simulink model "UAV_UGV_Coop"  (R2026a)
settings: Solver=ode4  StopTime=650  FixedStep=1e-3  MaxStep=0.001  MinStep=1e-6
PreLoadFcn:
  | % Caricamento automatico di tutte le variabili salvate
  | 
  | load('MappaEdifici.mat');
  | load('WaypointData.mat');
  | load('MappaGroundTruth.mat');
  | load('MappaScoperta_Altis.mat');
  | load('Percoso_UGV.mat');
  | load('UAV_x_d.mat');
  | load('UAV_x_r.mat');
  | load('UAV_y_d.mat');
  | load('UAV_y_r.mat');
  | load('UAV_z_d.mat');
  | load('UAV_z_r.mat');
  | load('UAV_phi_d.mat');
  | load('UAV_phi_r.mat');
  | load('UAV_theta_d.mat');
  | load('UAV_theta_r.mat');
  | load('UGV_x_d.mat');
  | load('UGV_x_r.mat');
  | load('UGV_y_d.mat');
  | load('UGV_y_r.mat');
  | load('UGV_psi.mat');
  | load('UGV_theta.mat');
  | load('A_fov.mat');
  | load('tout.mat');
model workspace: external: MAT-File MappaGroundTruth.mat (data not in the file)
undefined symbols (not defined in the file): MAPPA_EDIFICI, MAPPA_GROUND_TRUTH
settings Model: Creator=adriano  LastModifiedBy=Salvatore

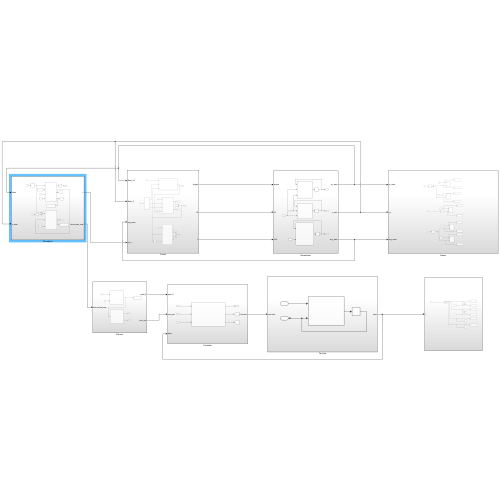
[thumbnail: Simulink's stored preview of the top-level diagram]
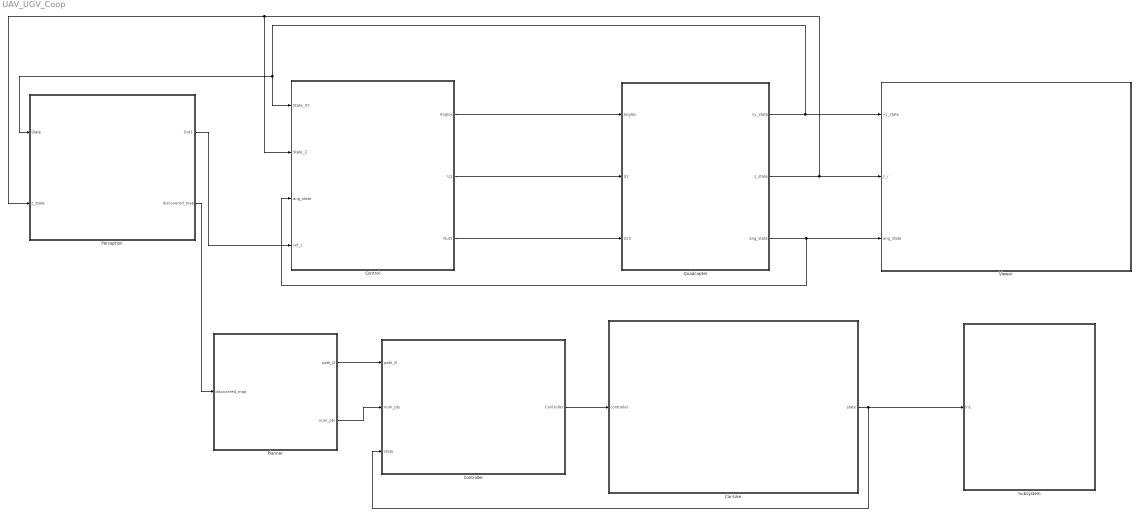
== system UAV_UGV_Coop ==
  Car-Like : Subsystem
  Control : Subsystem
  Controller : Subsystem
  Perception : Subsystem
  Planner : Subsystem
  Quadcopter : Subsystem
  Subsystem : Subsystem
  Viewer : Subsystem
  wires:
  Quadcopter/2(z_state) -> Control/2(State_Z), Perception/2(z_state), Viewer/2(z_r)
  Perception/1(Out1) -> Control/4(ref_z)
  Quadcopter/1(xy_state) -> Control/1(State_XY), Perception/1(State), Viewer/1(xy_state)
  Control/2(U1) -> Quadcopter/2(U1)
  Quadcopter/3(ang_state) -> Viewer/3(ang_state), Control/3(ang_state)
  Control/1(Angles) -> Quadcopter/1(angles)
  Control/3(Out1) -> Quadcopter/3(U23)
  Perception/2(discovered_map) -> Planner/1(discovered_map)
  Planner/1(path_D) -> Controller/1(path_D)
  Planner/2(num_pts) -> Controller/2(num_pts)
  Controller/1(Controller) -> Car-Like/1(controller)
  Car-Like/1(state) -> Controller/3(state), Subsystem/1(In1)

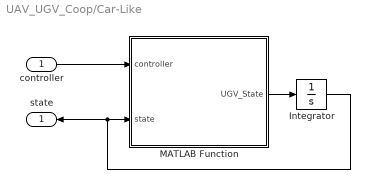
== system UAV_UGV_Coop/Car-Like ==
  controller : Inport
  Integrator : Integrator  InitialCondition=[17.0; 155.0; 0.0; 0.0]
  MATLAB Function : MATLAB Function  TreatAsAtomicUnit=on
  state : Outport
  wires:
  MATLAB Function/1(UGV_State) -> Integrator/1
  Integrator/1 -> MATLAB Function/2(state), state/1
  controller/1 -> MATLAB Function/1(controller)

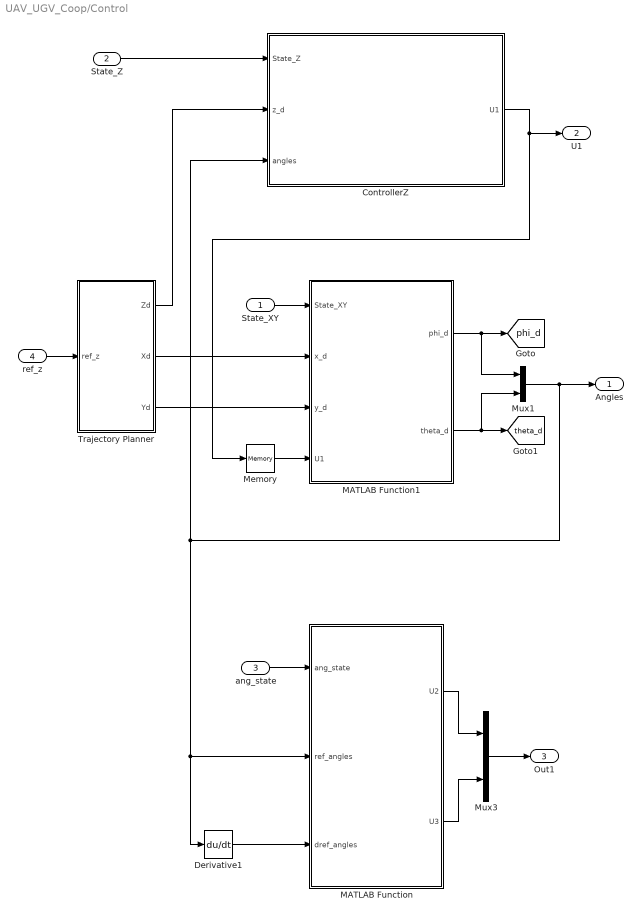
== system UAV_UGV_Coop/Control ==
  State_XY : Inport
  State_Z : Inport  Port=2
  ang_state : Inport  Port=3
  ref_z : Inport  Port=4
  ControllerZ : Subsystem
  Derivative1 : Derivative
  MATLAB Function : MATLAB Function  TreatAsAtomicUnit=on
  MATLAB Function1 : MATLAB Function  TreatAsAtomicUnit=on
  Memory : Memory
  Mux1 : Mux  Inputs=2
  Mux3 : Mux  Inputs=2
  Trajectory Planner : Subsystem
  Angles : Outport
  U1 : Outport  Port=2
  Out1 : Outport  Port=3
  tag scope: phi_d=global, theta_d=global
  wires:
  ref_z/1 -> Trajectory Planner/1(ref_z)
  State_Z/1 -> ControllerZ/1(State_Z)
  Trajectory Planner/1(Zd) -> ControllerZ/2(z_d)
  ControllerZ/1(U1) -> U1/1, Memory/1
  State_XY/1 -> MATLAB Function1/1(State_XY)
  ang_state/1 -> MATLAB Function/1(ang_state)
  Mux1/1 -> ControllerZ/3(angles), MATLAB Function/2(ref_angles), Derivative1/1, Angles/1
  MATLAB Function/1(U2) -> Mux3/1
  MATLAB Function/2(U3) -> Mux3/2
  Mux3/1 -> Out1/1
  Memory/1 -> MATLAB Function1/4(U1)
  MATLAB Function1/2(theta_d) -> [theta_d], Mux1/2
  MATLAB Function1/1(phi_d) -> [phi_d], Mux1/1
  Derivative1/1 -> MATLAB Function/3(dref_angles)
  Trajectory Planner/2(Xd) -> MATLAB Function1/2(x_d)
  Trajectory Planner/3(Yd) -> MATLAB Function1/3(y_d)

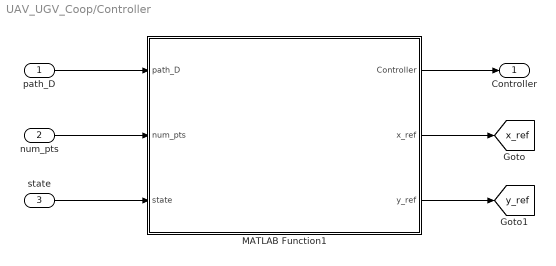
== system UAV_UGV_Coop/Controller ==
  path_D : Inport
  num_pts : Inport  Port=2
  state : Inport  Port=3
  MATLAB Function1 : MATLAB Function  TreatAsAtomicUnit=on
  Controller : Outport
  tag scope: x_ref=global, y_ref=global
  wires:
  state/1 -> MATLAB Function1/3(state)
  path_D/1 -> MATLAB Function1/1(path_D)
  MATLAB Function1/1(Controller) -> Controller/1
  num_pts/1 -> MATLAB Function1/2(num_pts)
  MATLAB Function1/2(x_ref) -> [x_ref]
  MATLAB Function1/3(y_ref) -> [y_ref]

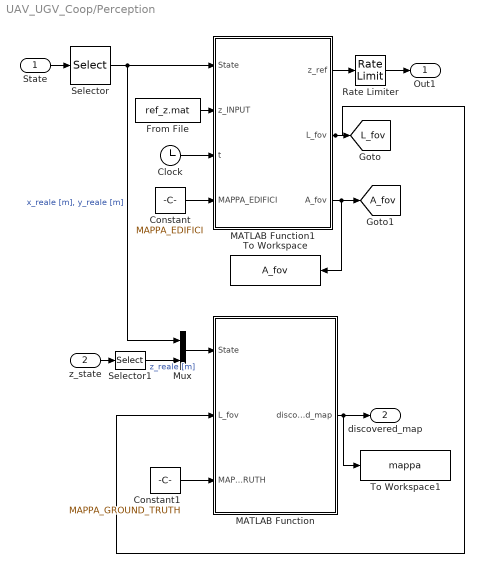
== system UAV_UGV_Coop/Perception ==
  State : Inport
  z_state : Inport  Port=2
  Clock : Clock
  Constant : Constant  Value=MAPPA_EDIFICI
  Constant1 : Constant  Value=MAPPA_GROUND_TRUTH
  From File : FromFile  FileName=ref_z.mat  SampleTime=0
  MATLAB Function : MATLAB Function  TreatAsAtomicUnit=on
  MATLAB Function1 : MATLAB Function  TreatAsAtomicUnit=on
  Mux : Mux  Inputs=2
  Rate Limiter : RateLimiter  SampleTimeMode=inherited
  Selector : Selector  InputPortWidth=4  IndexOptions=Index vector (dialog)  Indices=[1 3]  OutputSizes=1
  Selector1 : Selector  InputPortWidth=2  IndexOptions=Index vector (dialog)  Indices=[1]  OutputSizes=1
  To Workspace : ToWorkspace  VariableName=A_fov  SaveFormat=Timeseries  SampleTime=-1
  To Workspace1 : ToWorkspace  VariableName=mappa  SaveFormat=Timeseries  SampleTime=-1
      settings: MaxDataPoints=1
  Out1 : Outport
  discovered_map : Outport  Port=2
  tag scope: A_fov=global, L_fov=global
  wires:
  MATLAB Function1/2(L_fov) -> MATLAB Function/2(L_fov), [L_fov]
  From File/1 -> MATLAB Function1/2(z_INPUT)
  Rate Limiter/1 -> Out1/1
  MATLAB Function1/3(A_fov) -> [A_fov], To Workspace/1
  MATLAB Function1/1(z_ref) -> Rate Limiter/1
  State/1 -> Selector/1
  Selector/1 -> MATLAB Function1/1(State), Mux/1  "x_reale [m], y_reale [m]"
  Clock/1 -> MATLAB Function1/3(t)
  Constant/1 -> MATLAB Function1/4(MAPPA_EDIFICI)
  z_state/1 -> Selector1/1
  Selector1/1 -> Mux/2  "z_reale [m]"
  Mux/1 -> MATLAB Function/1(State)
  Constant1/1 -> MATLAB Function/3(MAPPA_GROUND_TRUTH)
  MATLAB Function/1(discovered_map) -> To Workspace1/1, discovered_map/1

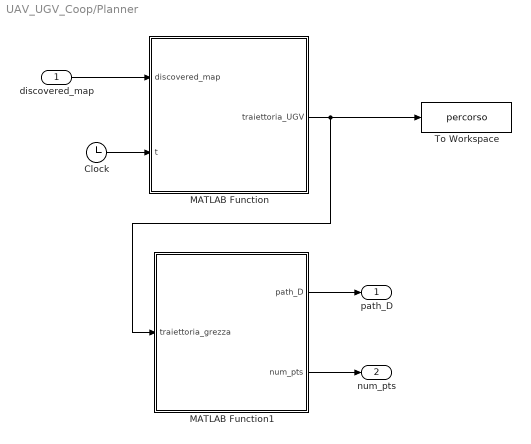
== system UAV_UGV_Coop/Planner ==
  discovered_map : Inport
  Clock : Clock
  MATLAB Function : MATLAB Function  TreatAsAtomicUnit=on
  MATLAB Function1 : MATLAB Function  TreatAsAtomicUnit=on
  To Workspace : ToWorkspace  VariableName=percorso  SaveFormat=Timeseries  SampleTime=-1
      settings: MaxDataPoints=1
  path_D : Outport
  num_pts : Outport  Port=2
  wires:
  Clock/1 -> MATLAB Function/2(t)
  MATLAB Function/1(traiettoria_UGV) -> To Workspace/1, MATLAB Function1/1(traiettoria_grezza)
  discovered_map/1 -> MATLAB Function/1(discovered_map)
  MATLAB Function1/1(path_D) -> path_D/1
  MATLAB Function1/2(num_pts) -> num_pts/1

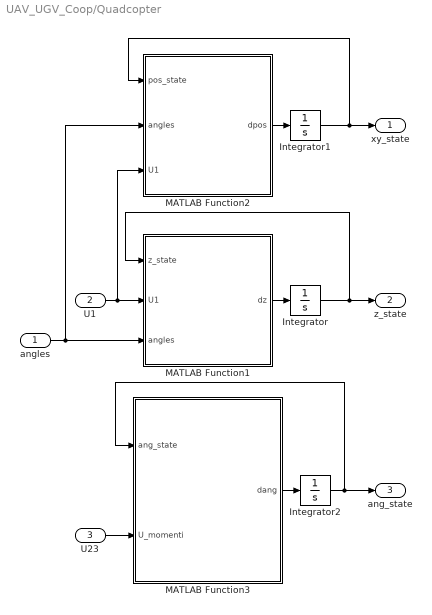
== system UAV_UGV_Coop/Quadcopter ==
  angles : Inport
  U1 : Inport  Port=2
  U23 : Inport  Port=3
  Integrator : Integrator
  Integrator1 : Integrator
  Integrator2 : Integrator
  MATLAB Function1 : MATLAB Function  TreatAsAtomicUnit=on
  MATLAB Function2 : MATLAB Function  TreatAsAtomicUnit=on
  MATLAB Function3 : MATLAB Function  TreatAsAtomicUnit=on
  xy_state : Outport
  z_state : Outport  Port=2
  ang_state : Outport  Port=3
  wires:
  MATLAB Function1/1(dz) -> Integrator/1
  Integrator/1 -> z_state/1, MATLAB Function1/1(z_state)
  angles/1 -> MATLAB Function2/2(angles), MATLAB Function1/3(angles)
  MATLAB Function2/1(dpos) -> Integrator1/1
  Integrator1/1 -> MATLAB Function2/1(pos_state), xy_state/1
  U1/1 -> MATLAB Function1/2(U1), MATLAB Function2/3(U1)
  MATLAB Function3/1(dang) -> Integrator2/1
  Integrator2/1 -> ang_state/1, MATLAB Function3/1(ang_state)
  U23/1 -> MATLAB Function3/2(U_momenti)

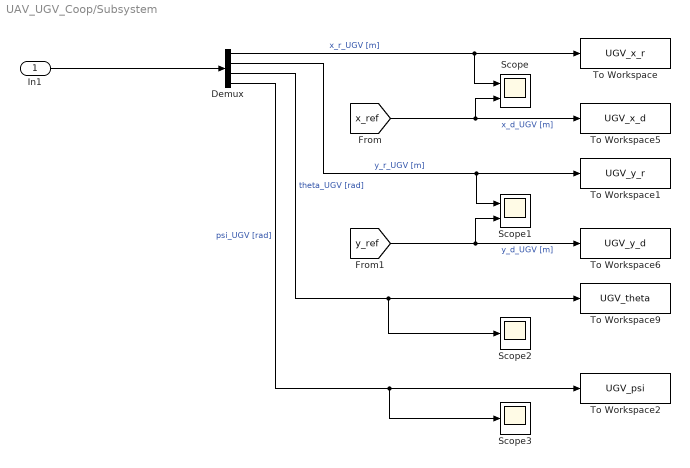
== system UAV_UGV_Coop/Subsystem ==
  In1 : Inport
  Demux : Demux
  Scope : Scope  NumInputPorts=2
      settings: ActiveDisplayYMinimum=-148.99376559580284  ActiveDisplayYMaximum=93.973074247656058  DataLoggingVariableName=ScopeData3
  Scope1 : Scope  NumInputPorts=2
      settings: ActiveDisplayYMinimum=31.631627910476041  ActiveDisplayYMaximum=174.01442830668728  DataLoggingVariableName=ScopeData4
  Scope2 : Scope
      settings: ActiveDisplayYMinimum=-4.4152539279638745  ActiveDisplayYMaximum=4.7250316272107744  DataLoggingVariableName=ScopeData5
  Scope3 : Scope
      settings: ActiveDisplayYMinimum=-0.76358154774750753  ActiveDisplayYMaximum=0.76358154774750753  DataLoggingVariableName=ScopeData6
  To Workspace : ToWorkspace  VariableName=UGV_x_r  SaveFormat=Timeseries  SampleTime=-1
  To Workspace1 : ToWorkspace  VariableName=UGV_y_r  SaveFormat=Timeseries  SampleTime=-1
  To Workspace2 : ToWorkspace  VariableName=UGV_psi  SaveFormat=Timeseries  SampleTime=-1
  To Workspace5 : ToWorkspace  VariableName=UGV_x_d  SaveFormat=Timeseries  SampleTime=-1
  To Workspace6 : ToWorkspace  VariableName=UGV_y_d  SaveFormat=Timeseries  SampleTime=-1
  To Workspace9 : ToWorkspace  VariableName=UGV_theta  SaveFormat=Timeseries  SampleTime=-1
  wires:
  Demux/2 -> Scope1/1, To Workspace1/1  "y_r_UGV [m]"
  Demux/1 -> Scope/1, To Workspace/1  "x_r_UGV [m]"
  [x_ref] -> Scope/2, To Workspace5/1  "x_d_UGV [m]"
  In1/1 -> Demux/1
  [y_ref] -> To Workspace6/1, Scope1/2  "y_d_UGV [m]"
  Demux/3 -> To Workspace9/1, Scope2/1  "theta_UGV [rad]"
  Demux/4 -> To Workspace2/1, Scope3/1  "psi_UGV [rad]"

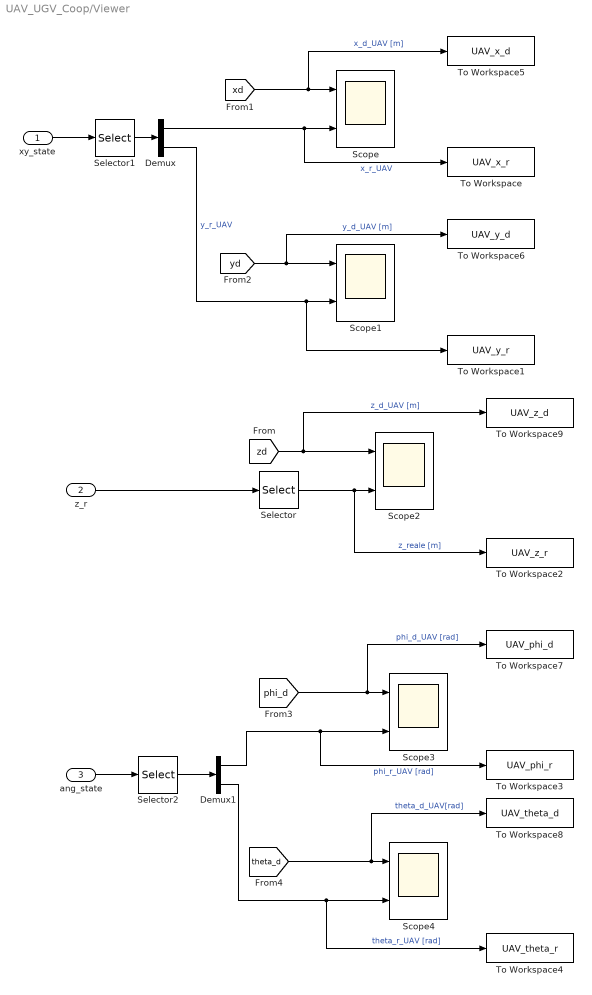
== system UAV_UGV_Coop/Viewer ==
  xy_state : Inport
  z_r : Inport  Port=2
  ang_state : Inport  Port=3
  Demux : Demux  Outputs=2
  Demux1 : Demux  Outputs=2
  Scope{,1..4} (5 alike) : Scope  NumInputPorts=2
      Scope settings: ActiveDisplayYMinimum=-242.12221615870175  ActiveDisplayYMaximum=120.41682539227989
      Scope1 settings: ActiveDisplayYMinimum=-23.676037505376105  ActiveDisplayYMaximum=207.37773635103918
      Scope2 settings: ActiveDisplayYMinimum=-7.8867312001852117  ActiveDisplayYMaximum=70.963722945541591  DataLoggingVariableName=ScopeData2
      Scope3 settings: ActiveDisplayYMinimum=-0.83331111959754556  ActiveDisplayYMaximum=0.72502273318878152  DataLoggingVariableName=ScopeData7
      Scope4 settings: ActiveDisplayYMinimum=-1  ActiveDisplayYMaximum=1  DataLoggingVariableName=ScopeData8
  Selector : Selector  InputPortWidth=2  IndexOptions=Index vector (dialog)  Indices=[1]  OutputSizes=1
  Selector1 : Selector  InputPortWidth=4  IndexOptions=Index vector (dialog)  Indices=[1 3]  OutputSizes=1
  Selector2 : Selector  InputPortWidth=4  IndexOptions=Index vector (dialog)  Indices=[1 3]  OutputSizes=1
  To Workspace : ToWorkspace  VariableName=UAV_x_r  SaveFormat=Timeseries  SampleTime=-1
  To Workspace1 : ToWorkspace  VariableName=UAV_y_r  SaveFormat=Timeseries  SampleTime=-1
  To Workspace2 : ToWorkspace  VariableName=UAV_z_r  SaveFormat=Timeseries  SampleTime=-1
  To Workspace3 : ToWorkspace  VariableName=UAV_phi_r  SaveFormat=Timeseries  SampleTime=-1
  To Workspace4 : ToWorkspace  VariableName=UAV_theta_r  SaveFormat=Timeseries  SampleTime=-1
  To Workspace5 : ToWorkspace  VariableName=UAV_x_d  SaveFormat=Timeseries  SampleTime=-1
  To Workspace6 : ToWorkspace  VariableName=UAV_y_d  SaveFormat=Timeseries  SampleTime=-1
  To Workspace7 : ToWorkspace  VariableName=UAV_phi_d  SaveFormat=Timeseries  SampleTime=-1
  To Workspace8 : ToWorkspace  VariableName=UAV_theta_d  SaveFormat=Timeseries  SampleTime=-1
  To Workspace9 : ToWorkspace  VariableName=UAV_z_d  SaveFormat=Timeseries  SampleTime=-1
  wires:
  Selector/1 -> To Workspace2/1, Scope2/2  "z_reale [m]"
  [yd] -> To Workspace6/1, Scope1/1  "y_d_UAV [m]"
  Demux/1 -> To Workspace/1, Scope/2  "x_r_UAV"
  [zd] -> To Workspace9/1, Scope2/1  "z_d_UAV [m]"
  [xd] -> To Workspace5/1, Scope/1  "x_d_UAV [m]"
  Demux/2 -> To Workspace1/1, Scope1/2  "y_r_UAV"
  z_r/1 -> Selector/1
  xy_state/1 -> Selector1/1
  Selector1/1 -> Demux/1
  ang_state/1 -> Selector2/1
  Selector2/1 -> Demux1/1
  Demux1/1 -> To Workspace3/1, Scope3/2  "phi_r_UAV [rad]"
  Demux1/2 -> To Workspace4/1, Scope4/2  "theta_r_UAV [rad]"
  [phi_d] -> To Workspace7/1, Scope3/1  "phi_d_UAV [rad]"
  [theta_d] -> To Workspace8/1, Scope4/1  "theta_d_UAV[rad]"

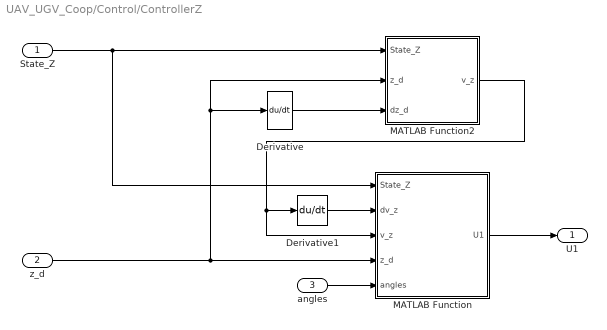
== system UAV_UGV_Coop/Control/ControllerZ ==
  State_Z : Inport
  z_d : Inport  Port=2
  angles : Inport  Port=3
  Derivative : Derivative
  Derivative1 : Derivative
  MATLAB Function : MATLAB Function  TreatAsAtomicUnit=on
  MATLAB Function2 : MATLAB Function  TreatAsAtomicUnit=on
  U1 : Outport
  wires:
  MATLAB Function/1(U1) -> U1/1
  State_Z/1 -> MATLAB Function/1(State_Z), MATLAB Function2/1(State_Z)
  z_d/1 -> MATLAB Function/4(z_d), MATLAB Function2/2(z_d), Derivative/1
  Derivative/1 -> MATLAB Function2/3(dz_d)
  MATLAB Function2/1(v_z) -> Derivative1/1, MATLAB Function/3(v_z)
  Derivative1/1 -> MATLAB Function/2(dv_z)
  angles/1 -> MATLAB Function/5(angles)

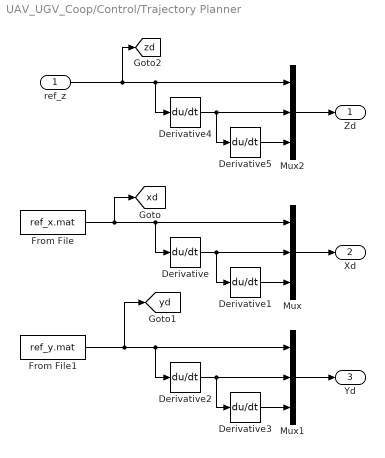
== system UAV_UGV_Coop/Control/Trajectory Planner ==
  ref_z : Inport
  Derivative{,1..5} (6 alike) : Derivative
  From File : FromFile  FileName=ref_x.mat  SampleTime=0
  From File1 : FromFile  FileName=ref_y.mat  SampleTime=0
  Mux : Mux  Inputs=3
  Mux1 : Mux  Inputs=3
  Mux2 : Mux  Inputs=3
  Zd : Outport
  Xd : Outport  Port=2
  Yd : Outport  Port=3
  tag scope: xd=global, yd=global, zd=global
  wires:
  Derivative/1 -> Derivative1/1, Mux/2
  Mux/1 -> Xd/1
  From File/1 -> [xd], Derivative/1, Mux/1
  Derivative1/1 -> Mux/3
  From File1/1 -> [yd], Derivative2/1, Mux1/1
  Derivative2/1 -> Derivative3/1, Mux1/2
  Derivative3/1 -> Mux1/3
  Mux1/1 -> Yd/1
  Derivative4/1 -> Derivative5/1, Mux2/2
  Derivative5/1 -> Mux2/3
  Mux2/1 -> Zd/1
  ref_z/1 -> [zd], Derivative4/1, Mux2/1

== matlab function UAV_UGV_Coop/Planner/MATLAB Function ==
  settings: updateMethod=DISCRETE
  data: discovered_map input; t input; traiettoria_UGV output double size=[3000 3]
function traiettoria_UGV = PrePianificazione_UGV(discovered_map, t)

% Buffer statico persistente per evitare ricalcoli continui
persistent traj_computed path_cached
if isempty(traj_computed)
    traj_computed = false;
    path_cached = zeros(3000, 3);
end

% Prima di 199s o se già calcolato, restituisci la memoria cache
if t < 199.0
    traiettoria_UGV = path_cached;
    return;
end

if traj_computed
    traiettoria_UGV = path_cached;
    return;
end

%% ================= ESECUZIONE SINGOLA APF (t = 199s) =================
n_rows = 251;
n_cols = 341;
x_min = -230.0; 
y_min = -36.0; 
res = 1.0;

wp = [  17.0, 155.0;   % START
       -50.0, 160.0;   % H1
      -115.0, 130.0;   % H2
        55.0,  45.0;   % H3
        70.0, 140.0;   % H4
      -125.0, 104.0;   % REFUEL
        17.0, 155.0];  % RIENTRO

ka = 1.5; 
kr = 35.0; 
rho0 = 5.0; 
dt = 0.5; 
ds_max = 1.5; 
r_box = 10;

pos = wp(1, :);
idx = 1;
path_cached(idx, 1:2) = pos;

for w = 1:size(wp, 1) - 1
    target = wp(w + 1, :);
    for step = 1:600
        if idx >= 3000
            break;
        end
        
        d = target - pos;
        dist = norm(d);
        if dist < 2.0
            break;
        end
        
        F = ka * d / dist;  % Forza attrattiva
        
        c0 = min(max(round((pos(1) - x_min) / res) + 1, 1), n_cols);
        r0 = min(max(round((pos(2) - y_min) / res) + 1, 1), n_rows);
        
        for r = max(1, r0 - r_box):min(n_rows, r0 + r_box)
            for c = max(1, c0 - r_box):min(n_cols, c0 + r_box)
                if discovered_map(r, c) > 0.5
                    od  = pos - [(c - 1) * res + x_min, (r - 1) * res + y_min];
                    do_ = norm(od);
                    if do_ > 0.01 && do_ < rho0
                        F = F + kr * (1 / do_ - 1 / rho0) / do_^2 * (od / do_);
                    end
                end
            end
        end
        
        nF = norm(F);
        if nF > 1e-4
            step_dir = F / nF;
        else
            step_dir = d / dist;
        end
        
        pos = pos + step_dir * min(ds_max, nF * dt);
        idx = idx + 1;
        path_cached(idx, 1:2) = pos;
    end
end

traj_computed = true; % Blocca l'esecuzione per tutti i passi temporali futuri
traiettoria_UGV = path_cached;
end

== matlab function UAV_UGV_Coop/Planner/MATLAB Function1 ==
  data: traiettoria_grezza input size=[3000 3]; path_D output double size=[3000, 3]; num_pts output
function [path_D, num_pts] = Pianificazione_UGV(traiettoria_grezza)

% Inizializzazione buffer statico 3000x3 Fixed-Size
path_D  = zeros(3000, 3);
num_pts = int32(0);
count   = int32(0);

% Scansione statica su 3000 righe (senza size dinamico)
for k = 1:3000
    val_x = traiettoria_grezza(k, 1);
    val_y = traiettoria_grezza(k, 2);
    
    % Se incontra il padding [0, 0] dopo il primo punto, interrompe
    if k > 1 && (val_x == 0.0 && val_y == 0.0)
        break;
    end
    
    if ~(val_x == 0.0 && val_y == 0.0)
        count = count + 1;
        path_D(count, 1) = val_x;
        path_D(count, 2) = val_y;
    end
end

num_pts = count;

== matlab function UAV_UGV_Coop/Car-Like/MATLAB Function ==
  data: controller input; UGV_State output; state input
function UGV_State = UGV_Kinematics(controller, state)
% Definizione dei parametri fisici
L = 2.5; % Dimensione interasse [m]

% Spacchettamento delle variabili di controllo
v = controller(1);
omega = controller(2);

% Spacchettamento degli stati
% state = [x; y; theta; psi]
theta = state(3); % Orientamento telaio [rad]
psi = state(4);   % Angolo di sterzo [rad]

% Modello cinematico con riferimento posteriore a trazione posteriore 
dx = cos(theta)*v;
dy = sin(theta)*v;
dtheta = 1/L*tan(psi)*v;
dpsi = omega;

% Uscita come derivata dello stato q_dot
UGV_State = [dx; dy; dtheta; dpsi];

== matlab function UAV_UGV_Coop/Controller/MATLAB Function1 ==
  settings: updateMethod=DISCRETE
  data: path_D input size=[3000 3]; num_pts input; state input; Controller output; x_ref output; y_ref output
function [Controller, x_ref, y_ref] = pure_pursuit_controller(path_D, num_pts, state)

%% Definizione Parametri
% Variabile persistente per l'integrale dell'errore
%% 1. Definizione Parametri e Inizializzazioni
%dt = 0.05;          % Passo temporale di campionamento [s]
d  = 6;           % Distanza nominale dal target d* [m]
v_cruise = 2.0;            % Velocita' di avanzamento nominale [m/s]

% Guadagni di Controllo (secondo Peter Corke)
%Kv   = 0.8;         % Guadagno proporzionale velocita'
%Ki   = 0.1;         % Guadagno integrale velocita'
Kh   = 1.2;         % Guadagno proporzionale di rotta (heading gain)
Kpsi = 6.0;         % Guadagno dell'attuatore di sterzo
psi_max = 35*pi/180;% Limite fisico di sterzo (35 gradi)

%% Spachettamento dello stato
x = state(1);
y = state(2);
theta = state(3);
psi = state(4);

% Variabile persistente per impedire al target di retrocedere
persistent last_idx
if isempty(last_idx)
    last_idx = int32(1);
end

% Variabile persistente per l'integrale dell'errore (con inizializzazione)
persistent e_integral
if isempty(e_integral)
    e_integral = 0.0;
end

% Se la pianificazione non ha ancora fornito punti, mantieni il veicolo fermo
if num_pts < 2
    Controller = [0.0; 0.0];
    x_ref = x;
    y_ref = y;
    return;
end



%% Ricerca Geometrica Monotona del Target Look-Ahead
% Avanzamento preventivo se il veicolo ha già superato/raggiunto il punto corrente
dist_current = sqrt((path_D(last_idx, 1) - x)^2 + (path_D(last_idx, 2) - y)^2);
if dist_current < 4.0 && last_idx < int32(num_pts - 10)
    last_idx = last_idx + int32(5); % Salta i punti già "consumati"
end

best_idx = last_idx;
min_diff = inf;

% Ricerca a partire da last_idx verso il termine del percorso
for k = last_idx:int32(num_pts)
    dist_k = sqrt((path_D(k, 1) - x)^2 + (path_D(k, 2) - y)^2);
    
    % Seleziona il primo punto utile a distanza >= d
    if dist_k >= d
        best_idx = k;
        break;
    end
    
    diff_val = abs(dist_k - d);
    if diff_val < min_diff
        min_diff = diff_val;
        best_idx = k;
    end
end

% Aggiorna l'indice persistente in modo strettamente monotono
last_idx = max(last_idx, best_idx);

% Emissione delle sole coordinate target [x_d; y_d]
x_d = path_D(best_idx, 1);
x_ref = x_d;
y_d = path_D(best_idx, 2);
y_ref = y_d;
%% Controllo di sterzatura

% Definizione dell'orientamento desiderato
theta_d = atan2(y_d - y, x_d - x); 
% Errore d'orientamento normalizzato
e_theta = theta_d - theta;
e_theta = atan2(sin(e_theta), cos(e_theta));
% Definizione dell'angolo di sterzo desiderato con saturazione
psi_d = Kh * e_theta; 
psi_d = min(max(psi_d, -psi_max), psi_max);
% Calcolo dell'ingresso di comando di sterzatura
omega_star = Kpsi * (psi_d - psi);

%% 5. Profilo di Velocità Longitudinale (Feedforward + Stop al Goal)
dist_goal = sqrt((path_D(num_pts, 1) - x)^2 + (path_D(num_pts, 2) - y)^2);

if dist_goal < 1.2
    % Arresto finale completato al traguardo
    v_star = 0.0;
    omega_star = -Kpsi * psi; % Raddrizza le ruote
elseif dist_goal < 6.0
    % Decelerazione lineare negli ultimi metri
    v_star = v_cruise * (dist_goal / 6.0);
    v_star = max(0.4, v_star);
else
    % Avanzamento a velocità nominale
    v_star = v_cruise;
end

%% 6. Vettore Uscita Comandi
Controller = [v_star; omega_star];
end

== matlab function UAV_UGV_Coop/Control/ControllerZ/MATLAB Function ==
  data: State_Z input; U1 output size=1; dv_z input; v_z input; z_d input; angles input
function U1 = controller2_Z(State_Z, dv_z, v_z, z_d, angles)
    %U1 = 0;
    k2_z = 5; % Guadagno Lyapunov Step 2
    m = 1.2;  % Massa UAV [kg]
    g = 9.81; % Gravità [m/s^2]
    
    z = State_Z(1);
    z_dot = State_Z(2);
    phi = angles(1);   % Roll
    theta = angles(2); % Pitch
    
    z1 = z - z_d;
    z2 = z_dot - v_z; % Errore sulla velocità verticale
    term = g + dv_z(1) - z1(1) - k2_z * z2(1);
    % Legge di controllo reale U1 (Spinta totale)
    % Cancella la gravità e garantisce dV/dt < 0
    U1 = (m / (cos(phi) * cos(theta))) * term;
end

== matlab function UAV_UGV_Coop/Control/ControllerZ/MATLAB Function2 ==
  data: State_Z input; v_z output; z_d input; dz_d input
function v_z = controller1_Z(State_Z, z_d, dz_d)
    k1_z = 2; % Guadagno Lyapunov Step 1
    
    z = State_Z(1);
    z1 = z - z_d; % Errore di quota
    
    % Variabile di controllo virtuale per z_dot
    v_z = dz_d - k1_z * z1;
end

== matlab function UAV_UGV_Coop/Perception/MATLAB Function1 ==
  data: State input; z_ref output; z_INPUT input; t input; MAPPA_EDIFICI input; L_fov output; A_fov output
function [z_ref, L_fov, A_fov] =  FOV_planner(State, z_INPUT, t, MAPPA_EDIFICI)
    % 1. Posizione attuale del drone
    x_drone = State(1);
    y_drone = State(2);
    
    % 2. Parametro FOV Telecamera (es. 60 gradi)
    fov_deg = 60;
    fov_rad = fov_deg * (pi / 180);
    
    % 3. Scansione di TUTTI gli edifici presenti nella mappa
    z_req_max = 0;
    num_edifici = size(MAPPA_EDIFICI, 1);
    
    for i = 1:num_edifici
        x_edificio   = MAPPA_EDIFICI(i, 1);
        y_edificio   = MAPPA_EDIFICI(i, 2);
        dim_edificio = MAPPA_EDIFICI(i, 3);
        
        % Distanza orizzontale dal centro dell'edificio
        dist = hypot(x_drone - x_edificio, y_drone - y_edificio);
        
        % Se il drone sta sorvolando l'edificio (o si trova dentro il suo raggio d'influenza)
        raggio_influenza = dim_edificio / 2 + 100; 
        
        if dist < raggio_influenza
            % Calcola la Z minima necessaria affinché l'impronta FOV contenga l'edificio
            z_min_necessaria = (dim_edificio * 1.70) / (2 * tan(fov_rad / 2));
            
            if z_min_necessaria > z_req_max
                z_req_max = z_min_necessaria;
            end
        end
    end
    
    % 4. Quota finale: garantisce la navigazione base o la quota di copertura completa
    z_ref = max(z_INPUT, z_req_max);
    % 5. CALCOLO DELLA CARATTERISTICA FOV (Lato inquadratura desiderato)
    % Calcoliamo l'impronta a terra generata dalla nuova quota z_ref
    L_fov = 2 * z_ref * tan(fov_rad / 2); 
    A_fov = L_fov^2;    
    % 2. Condizione di Atterraggio Finale:
    % tolleranza di 50 cm (0.5m) e attivazione solo a fine missione
    if (abs(x_drone) < 0.5 && abs(y_drone) < 0.5 && t > 0)
        z_ref = z_INPUT; % Assegna la discesa a terra fino a 0m
    else
        z_ref = max(z_INPUT, z_req_max); % In tutto il resto della mappa garantisce la massima quota FOV
    end
end

== matlab function UAV_UGV_Coop/Quadcopter/MATLAB Function1 ==
  data: z_state input size=2; dz output; U1 input; angles input size=2
function dz = sistema_dinamico_Z(z_state, U1, angles)
    % z_state = [z; z_dot]
    z = z_state(1);
    z_dot = z_state(2);
    phi = angles(1);   % Roll reale
    theta = angles(2); % Pitch reale
    m = 1.2;               % Massa drone [kg]
    g = 9.81;              % Gravità [m/s^2]
    
    dz1 = z_dot;
    dz2 = -g + (cos(phi)*cos(theta)/m) * U1;
    
    dz = [dz1; dz2];
end

== matlab function UAV_UGV_Coop/Quadcopter/MATLAB Function2 ==
  data: pos_state input; dpos output; angles input; U1 input
function dpos = sistema_dinamico_XY(pos_state, angles, U1)
    % pos_state = [x; x_dot; y; y_dot]
    % angles    = [phi; theta]  (gli angoli usciti da ControllerXY)
    % U1        = spinta reale proveniente da ControllerZ
    
    m = 1.2; % Massa del drone [kg]
    
    phi   = angles(1);
    theta = angles(2);
    
    x_dot = pos_state(2);
    y_dot = pos_state(4);

    % Accelerazioni REALI sul piano XY generate da inclinazione e spinta:
    x_ddot = (U1 / m) * sin(theta);  % Inclinazione di pitch genera forza lungo X     
    y_ddot = -(U1 / m) * sin(phi)*cos(theta);   % Inclinazione di roll genera forza lungo Y    


    
    dpos = [x_dot; x_ddot; y_dot; y_ddot];
end

== matlab function UAV_UGV_Coop/Quadcopter/MATLAB Function3 ==
  data: ang_state input; dang output size=4; U_momenti input
function dang = sistema_dinamico_Attitude(ang_state, U_momenti)
% ang_state = [phi; p; theta; q]
% U_momenti = [U2; U3]
Ix = 0.01; Iy = 0.01; % Inerzie UAV

phi   = ang_state(1);
p     = ang_state(2);
theta = ang_state(3);
q     = ang_state(4);

U2 = U_momenti(1);
U3 = U_momenti(2);

% Cinematica corretta: q guida dtheta, p guida dphi
dphi   = p; 
dp     = (1/Ix) * U2;
dtheta = q; 
dq     = (1/Iy) * U3;

dang = [dphi; dp; dtheta; dq];
end

== matlab function UAV_UGV_Coop/Control/MATLAB Function1 ==
  data: phi_d output; theta_d output; State_XY input; x_d input; y_d input; U1 input
function [phi_d, theta_d] = controller_XY(State_XY, x_d, y_d, U1)
    % Guadagni di controllo Backstepping
    k1_x = 1.8; k2_x = 5.5;
    k1_y = 1.8; k2_y = 5.5;
    m = 1.2;
    
    % --- 1. SPACCHETTAMENTO RIFERIMENTI (Target) ---
    % x_d e y_d sono vettori a 3 elementi: [posizione, velocità, accelerazione]
    xd   = x_d(1);   dxd  = x_d(2);   ddxd = x_d(3);
    yd   = y_d(1);   dyd  = y_d(2);   ddyd = y_d(3);
    
    % --- 2. SPACCHETTAMENTO STATO REALE (Misurato) ---
    x     = State_XY(1); 
    x_dot = State_XY(2);
    y     = State_XY(3); 
    y_dot = State_XY(4);
    
    % --- 3. STEP 1 BACKSTEPPING: Errori di posizione e Velocità Virtuali ---
    ex = xd - x;
    ey = yd - y;
    
    % Velocità virtuali desiderate
    VirtVel_x = dxd + k1_x * ex;
    VirtVel_y = dyd + k1_y * ey;
    
    % --- 4. STEP 2 BACKSTEPPING: Derivate delle velocità virtuali ed Errori di velocità ---
    % Derivata temporale della velocità virtuale
    dVirtVel_x = ddxd + k1_x * (dxd - x_dot);
    dVirtVel_y = ddyd + k1_y * (dyd - y_dot);
    
    % Errori sulle velocità
    zx2 = VirtVel_x - x_dot;
    zy2 = VirtVel_y - y_dot;
    
    % Accelerazioni virtuali richieste (u_x, u_y)
    u_x = dVirtVel_x + ex + k2_x * zx2;
    u_y = dVirtVel_y + ey + k2_y * zy2;
    
    % --- 5. CONVERSIONE IN ANGOLI DESIDERATI ---
    % Calcolo NON LINEARE esatto degli angoli (con protezione matematica del dominio [-1, 1])
    theta_d = asin( min(max( (m / U1) * u_x, -1), 1) );

    % Compensazione attiva dell'accoppiamento di beccheggio sulla dinamica di rollio
    phi_d   = asin( min(max( -(m / (U1 * cos(theta_d))) * u_y, -1), 1) );

    % --- 6. SATURAZIONE DI SICUREZZA SUGLI ANGOLI (30 GRADI) ---
    max_ang = 30 * (pi / 180); % 0.5236 rad
    
    phi_d   = min(max(phi_d, -max_ang), max_ang);    
    theta_d = min(max(theta_d, -max_ang), max_ang);
end

== matlab function UAV_UGV_Coop/Control/MATLAB Function ==
  data: ang_state input; U2 output; ref_angles input; dref_angles input; U3 output
function [U2, U3] = Controller_Attitude(ang_state, ref_angles, dref_angles)
        % ang_state   = [phi; p; theta; q]
        % ref_angles  = [phi_d; theta_d]
        % dref_angles = [dphi_d; dtheta_d]

        k1_phi = 10; k2_phi = 15;
        k1_th  = 10; k2_th  = 15;

        Ix = 0.01; Iy = 0.01;

        phi   = ang_state(1); p = ang_state(2);
        theta = ang_state(3); q = ang_state(4);

        phi_d   = ref_angles(1);  theta_d  = ref_angles(2);
        dphi_d  = dref_angles(1); dtheta_d = dref_angles(2);

        % --- STEP 1: Cinematica reale ---
        dphi   = p;
        dtheta = q;

        % --- STEP 2: Velocità virtuali (Backstepping / Lyapunov Step 1) ---
        e_phi   = phi - phi_d;
        e_theta = theta - theta_d;

        p_v = dphi_d   - k1_phi * e_phi;
        q_v = dtheta_d - k1_th  * e_theta;

        % --- STEP 3: Accelerazioni virtuali ---
        dp_v = -k1_phi * (dphi - dphi_d);
        dq_v = -k1_th  * (dtheta - dtheta_d);

        % --- STEP 4: Errori di velocità angolare (Lyapunov Step 2) ---
        e2_p = p - p_v;
        e2_q = q - q_v;

        max_torque = 2.0; 

        U2 = Ix * (dp_v - e_phi   - k2_phi * e2_p);
        U3 = Iy * (dq_v - e_theta - k2_th  * e2_q);

        % Saturazione
        U2 = min(max(U2, -max_torque), max_torque);
        U3 = min(max(U3, -max_torque), max_torque);
    end

== matlab function UAV_UGV_Coop/Perception/MATLAB Function ==
  settings: updateMethod=DISCRETE
  data: State input; discovered_map output; L_fov input; MAPPA_GROUND_TRUTH input
function discovered_map = UAV_Mapper(State, L_fov, MAPPA_GROUND_TRUTH)
% UAV_Mapper: Scansiona il Digital Twin reale tramite il FOV della telecamera
% e popola progressivamente la mappa di occupazione (discovered_map).

% --- COSTANTI GRIGLIA LOCALE ---
x_min = -230; % [m]
y_min = -36;  % [m]
res   = 1.0;  % [m/cella]

[num_rows, num_cols] = size(MAPPA_GROUND_TRUTH);

% --- MEMORIA PERSISTENTE (Mappa scoperta dal drone) ---
persistent map_discovered
if isempty(map_discovered)
    map_discovered = zeros(num_rows, num_cols); % Inizialmente completamente buia (0)
end

% --- POSIZIONE UAV E IMPRONTA FOV ---
x_d = State(1);
y_d = State(2);
half_fov = L_fov / 2;

% Limiti dell'impronta della telecamera a terra (rettangolo FOV)
fov_x_min = x_d - half_fov;
fov_x_max = x_d + half_fov;
fov_y_min = y_d - half_fov;
fov_y_max = y_d + half_fov;

% Conversione coordinate metriche FOV in indici di matrice (righe/colonne)
c_min = max(1, min(num_cols, round((fov_x_min - x_min) / res) + 1));
c_max = max(1, min(num_cols, round((fov_x_max - x_min) / res) + 1));
r_min = max(1, min(num_rows, round((fov_y_min - y_min) / res) + 1));
r_max = max(1, min(num_rows, round((fov_y_max - y_min) / res) + 1));

% --- SCANSIONE E SVELAMENTO DIGITAL TWIN ---
% Estrae la porzione visibile dalla Ground Truth ed esegue la fusione (OR logico)
map_discovered(r_min:r_max, c_min:c_max) = ...
    max(map_discovered(r_min:r_max, c_min:c_max), ...
    MAPPA_GROUND_TRUTH(r_min:r_max, c_min:c_max));

% Output aggiornato ad ogni passo di simulazione
discovered_map = map_discovered;
